simulink model "Controller_Pioneer3DXAssembly"  (R2013b)
settings: Solver=ode45  StartTime=0.0  StopTime=200  RelTol=1e-3
InitFcn:
  | load WorldLUTData.mat
  | r = 0.095; %Wheel radius
  | b = 0.33; %Wheel base
values from neighbouring files (symbols this model uses):
  World_LUT = [1 1 1 1 1 1 1 1 1 1 1 1 ... (24014001 elements, 2001x12001)]    [WorldLUTData.mat]
undefined symbols (not defined in the file or in its folder): X, Y, Z
libraries: sm_lib x35, nesl_utility x19, fl_lib x6, vrlib x2
(part 2 of 2)

== system Controller_Pioneer3DXAssembly/SM-->SL3D Interface/RWSL3D/Subsystem ==
  PS-Simulink Converter : nesl_utility/PS-Simulink Converter  PhysicalDomain=network_engine_domain  SubClassName=ps_output  LeftPortType=input  RightPortType=output  PseudoPeriodic=off  Frequencies=[]  Unit=1  AffineConversion=off
  Conn1 : PMIOPort  Port=1  Side=Left
  Omega_z : Outport
  wires:
  PS-Simulink Converter/1 -> Omega_z/1
  connections:
  Conn1/RConn1 -- PS-Simulink Converter/LConn1

== stateflow chart Controller_Pioneer3DXAssembly/Control Algorithm ==
  state Modes
    en,du:
    frontSensors = SonarSensors(4:5) < SensorRanges(4:5);
    leftMostSensors = [SonarSensors(1)] < SensorRanges(1);
    leftMiddleSensors = [SonarSensors(2:3)] < SensorRanges(2:3);
    rightMiddleSensors = [SonarSensors(6:7)] < SensorRanges(6:7);
    rightMostSensors = [SonarSensors(8) ]< SensorRanges(8);
    state ReverseABit
      en,du:
      RightVel = -v0;
      LeftVel = -v0;
    state GoStraight
      en,du:
      RightVel = v0;
      LeftVel = v0;
    state DetermineLeftRight
    state TurnRightInPlace
      du :
      RightVel = -v0;
      LeftVel = v0;
    state TurnLeftInPlace
      du :
      RightVel = v0;
      LeftVel = -v0;
    state TurnRightTight
      du :
      RightVel = v0/5;
      LeftVel = v0;
    state TurnLeftTight
      du :
      RightVel = v0;
      LeftVel = v0/5;
    state TurnRightWide
      du:
      RightVel = v0/2;
      LeftVel = v0;
    state TurnLeftWide
      du :
      RightVel = v0;
      LeftVel = v0/2;
    (default) -> ReverseABit
    ReverseABit -> GoStraight : after(3,sec)
    TurnRightWide -> GoStraight : [all(leftMostSensors<1)]
    GoStraight -> TurnRightWide [order 4] : [any(leftMostSensors>0)]
    TurnRightTight -> GoStraight : [all(leftMiddleSensors<1)]
    GoStraight -> TurnRightTight [order 2] : [any(leftMiddleSensors>0)]
    TurnRightInPlace -> GoStraight : [all(frontSensors<1)]
    GoStraight -> DetermineLeftRight [order 1] : [any(frontSensors>0)]
    TurnLeftInPlace -> GoStraight : [all(frontSensors<1)]
    TurnLeftTight -> GoStraight : [all(rightMiddleSensors<1)]
    GoStraight -> TurnLeftTight [order 3] : [any(rightMiddleSensors>0)]
    TurnLeftWide -> GoStraight : [all(rightMostSensors<1)]
    GoStraight -> TurnLeftWide [order 5] : [any(rightMostSensors>0)]
    DetermineLeftRight -> TurnRightInPlace [order 1] : [SonarSensors(4)>SonarSensors(5)]
    DetermineLeftRight -> TurnLeftInPlace [order 2] : %default
  data: LeftVel output; RightVel output; SonarSensors input; frontSensors local; SensorRanges input; v0 parameter; leftMostSensors local; leftMiddleSensors local; rightMostSensors local; rightMiddleSensors local

== matlab function Controller_Pioneer3DXAssembly/Virtual Sensors Subsystem/MATLAB Function ==
  data: x input; y input; rotMat input; xRange output; yRange output; r_range parameter size=8
function [xRange, yRange] = getVirtualBox(x,y,rotMat, r_range)
%#codegen
%% Dimensions
r_com = 0.27/2;%Radius of the SONAR arc in 'm'
r_range_m = r_range/1000;
% r_range = 0.5;%Radius of SONAR range in 'm'
r_b = r_com + r_range_m;%Back SONAR arc radius
yb_b = 0.18;%Shift in Y axis from COM

r_f = r_com + r_range_m;%Front SONAR arc radius, same as back in our case
yb_f = 0.09;%Shift in Y axis from COM

SensorPos = zeros(16,2);
SensorPosNew = zeros(16,3);
%% FRONT SENSORS
SensorPos(1,:) = [r_f(1)*sind(-90), r_f(1)*cosd(-90)+yb_f];
SensorPos(8,:) = [r_f(8)*sind(90), r_f(8)*cosd(90)+yb_f];

%Remaining front sensors
i = 2;
for theta = -50:20:50
    SensorPos(i,:) = [r_f(i)*sind(theta), r_f(i)*cosd(theta)+yb_f];
    i = i+1;
end

%% BACK SENSORS
SensorPos(9,:) = [r_b(1)*sind(90), r_b(1)*cosd(90)-yb_b];
SensorPos(16,:) = [r_b(8)*sind(-90), r_b(8)*cosd(-90)-yb_b];

%Remaining back sensors
i = 10;
for theta = -50:20:50
    SensorPos(i,:) = [-r_b(i-8)*sind(theta), -r_b(i-8)*cosd(theta)-yb_b];
    i = i+1;
end
rotZ90 = [0 -1 0; 1 0 0; 0 0 1];
rotMatNew = rotMat * rotZ90;
for i = 1:16
    SensorPosNew(i,:) = (rotMatNew*[SensorPos(i,:)';0] + [x; y;0])';
end

xRange = SensorPosNew(:,1);%Inp(:,1);
yRange = SensorPosNew(:,2);%-Inp(:,2);
